simulink model "ECGGENDemo"  (Simulink 4.00)
settings: Solver=FixedStepDiscrete  StartTime=0.0  StopTime=4096  RelTol=1e-3
libraries: bus_alteradspbuilder x10, store_alteradspbuilder x10, arithm_alteradspbuilder x2
settings Model: LastModifiedBy=igors

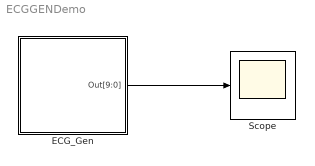
== system ECGGENDemo ==
  ECG_Gen : Subsystem  AncestorBlock=ALTELINK/AltLab/HDL SubSystem
      settings: RTWFcnNameOpts=Auto  RTWFileNameOpts=Auto
      mask Type: SubSystem AlteraBlockSet
  Scope : Scope
      settings: TimeRange=4096  YMin=-600  YMax=400  SaveToWorkspace=off  SaveName=ScopeData  LimitDataPoints=on  MaxDataPoints=5000
  wires:
  ECG_Gen/1(Out[9:0]) -> Scope/1

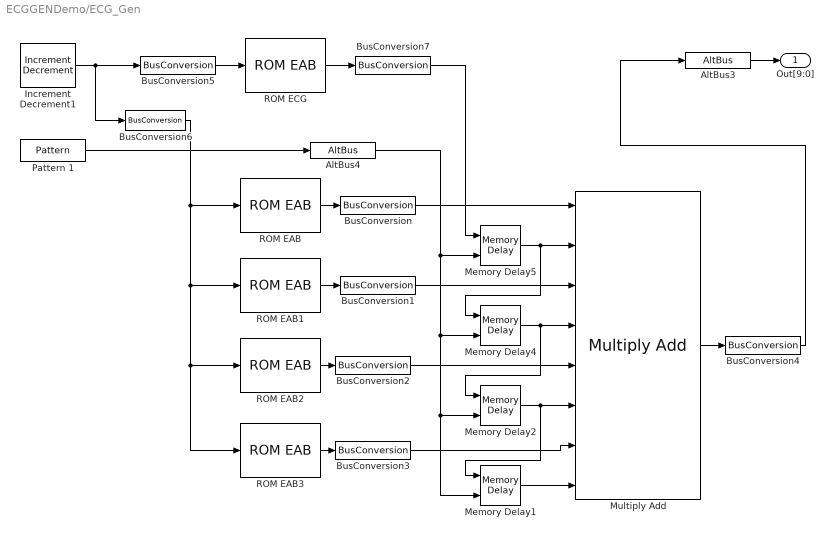
== system ECGGENDemo/ECG_Gen ==
  AltBus3 : bus_alteradspbuilder/AltBus  Description=Sign Binary Fractionnal  sgn=Signed Integer  nodetype=Output Port  bwl=10  bwr=8  sat=off  rnd=off  bp=off  mask_cst=0  LocPin=any  cst=0  modulename=AltBus3  nSgCpl=0
  AltBus4 : bus_alteradspbuilder/AltBus  Description=Sign Binary Fractionnal  sgn=Single Bit  nodetype=Input Port  bwl=1  bwr=0  sat=off  rnd=off  bp=off  mask_cst=0  LocPin=any  cst=0  modulename=AltBus4  nSgCpl=0
  BusConversion{,1..3,7} (5 alike) : bus_alteradspbuilder/BusConversion  Inputs=Signed Integer  bwl=16  bwr=8  Outputs=Signed Integer  obwl=14  obwr=0  msb=13  lsb=0  rnd=off  sat=off
  BusConversion4 : bus_alteradspbuilder/BusConversion  Inputs=Signed Integer  bwl=26  bwr=8  Outputs=Signed Integer  obwl=10  obwr=0  msb=20  lsb=11  rnd=off  sat=off
  BusConversion5 : bus_alteradspbuilder/BusConversion  Inputs=Signed Integer  bwl=9  bwr=8  Outputs=Unsigned Integer  obwl=6  obwr=0  msb=8  lsb=4  rnd=off  sat=off
  BusConversion6 : bus_alteradspbuilder/BusConversion  Inputs=Signed Integer  bwl=9  bwr=8  Outputs=Unsigned Integer  obwl=4  obwr=0  msb=3  lsb=0  rnd=off  sat=off
  Increment Decrement1 : arithm_alteradspbuilder/Increment Decrement  BusType=Signed Integer  bwl=9  bwr=4  direction=Increment  cst=0  clken=off  ntsamp=1  MaskValue=1
  Memory Delay{1..2,4..5} (4 alike) : store_alteradspbuilder/Memory Delay  bwaddr=1  depth=1  cst=off  clken=on  eab=on  vDepthAltr=1
  Multiply Add : arithm_alteradspbuilder/Multiply Add  depth=4  BusType=Signed Integer  bwl=14  bwr=0  direction=Add Add  pipeline=No Register  clken=off  eab=off  cst=off  Constantvalues=[1 1 1 1]  gain=[1.000000,1.000000,1.000000,1.000000]
  Pattern 1 : store_alteradspbuilder/Pattern  Priority=28  clken=off  ntsamp=1  MaskValue=0000000000000001
  ROM EAB : store_alteradspbuilder/ROM EAB  BusType=Signed Integer  bwl=16  bwr=0  bwaddr=4  Inputs=spl01604.hex  MaskValue=1
  ROM EAB1 : store_alteradspbuilder/ROM EAB  BusType=Signed Integer  bwl=16  bwr=0  bwaddr=4  Inputs=spl01603.hex  MaskValue=1
  ROM EAB2 : store_alteradspbuilder/ROM EAB  BusType=Signed Integer  bwl=16  bwr=0  bwaddr=4  Inputs=spl01602.hex  MaskValue=1
  ROM EAB3 : store_alteradspbuilder/ROM EAB  BusType=Signed Integer  bwl=16  bwr=0  bwaddr=4  Inputs=spl01601.hex  MaskValue=1
  ROM ECG : store_alteradspbuilder/ROM EAB  BusType=Signed Integer  bwl=16  bwr=0  bwaddr=5  Inputs=ecg32.hex  MaskValue=1
  Out[9:0] : Outport  Port=1
  wires:
  AltBus3/1 -> Out[9:0]/1
  BusConversion6/1 -> ROM EAB/1, ROM EAB1/1, ROM EAB2/1, ROM EAB3/1
  ROM EAB/1 -> BusConversion/1
  ROM EAB1/1 -> BusConversion1/1
  ROM EAB2/1 -> BusConversion2/1
  ROM EAB3/1 -> BusConversion3/1
  BusConversion/1 -> Multiply Add/1
  BusConversion1/1 -> Multiply Add/3
  BusConversion2/1 -> Multiply Add/5
  BusConversion3/1 -> Multiply Add/7
  Multiply Add/1 -> BusConversion4/1
  Memory Delay5/1 -> Multiply Add/2, Memory Delay4/1
  Memory Delay4/1 -> Multiply Add/4, Memory Delay2/1
  Memory Delay2/1 -> Multiply Add/6, Memory Delay1/1
  Memory Delay1/1 -> Multiply Add/8
  Pattern 1/1 -> AltBus4/1
  BusConversion4/1 -> AltBus3/1
  AltBus4/1 -> Memory Delay5/2, Memory Delay4/2, Memory Delay1/2, Memory Delay2/2
  ROM ECG/1 -> BusConversion7/1
  BusConversion5/1 -> ROM ECG/1
  Increment Decrement1/1 -> BusConversion5/1, BusConversion6/1
  BusConversion7/1 -> Memory Delay5/1
